simulink model "walkingRobotRL3D"  (R2020b)
settings: Solver=ode23t  StartTime=0.0  StopTime=Tf  RelTol=1e-2  EnableMultiTasking=on
PreLoadFcn:
  | robotParametersRL
undefined symbols (not defined in the file): agent, ankleD_pitch_jointMAX, ankleD_pitch_jointMIN, ankleD_roll_jointMAX, ankleD_roll_jointMIN, ankleI_pitch_jointMAX, ankleI_pitch_jointMIN, ankleI_roll_jointMAX, ankleI_roll_jointMIN, getSampleTime, height_plane, hipD_pitch_jointMAX, hipD_pitch_jointMIN, hipD_roll_jointMAX, hipD_roll_jointMIN, hipI_pitch_jointMAX, hipI_pitch_jointMIN, hipI_roll_jointMAX, hipI_roll_jointMIN, init_angs_L, init_angs_R, init_height, joint_damping, joint_limit_damping, joint_limit_stiffness, joint_stiffness, kneeD_jointMAX, kneeD_jointMIN, kneeI_jointMAX, kneeI_jointMIN, lower_leg_I0, lower_leg_length, lower_leg_mass, lower_leg_x, lower_leg_y, muscle_nominal_length, p10_ankleD_roll, plane_x, plane_y, regulator_type, tau, Tf, torso_height, torso_length, torso_offset_x, torso_offset_z, torso_width, torso_x, torso_y, torso_z, Ts, upper_leg_I0, upper_leg_length, upper_leg_mass, upper_leg_x, upper_leg_y, v10_ankleD_pitch, v10_ankleD_roll, v10_ankleI_pitch, v10_ankleI_roll ... (+41)
libraries: sm_lib x222, simulink x183, nesl_utility x130, walkingRobotUtils x69, rllib x2
(part 21 of 24)

== matlab function walkingRobotRL3D/Walking Robot/DYNAMIC MODEL OF PAM FOR RIGHT LEG/Dynamic Model Antagonisitic PAM2/Proportional Regulator (Muscles 1) ==
  data: V1 input; reg_type input; p1 output
% Author: Eduardo Reyero Ibáñez
% Descrition: In this file it will be implemented the required input for the PAM
function p1  = propReg(V1,reg_type)
%% Proportional pressure regulators VPPM
%Range of Voltage
minVoltage = 0;
maxVoltage = 7.98; % This voltage provide 8 bar of pressure with regulator type 1
p1 = zeros(1,1);
%Select regulartor type
%reg_type = 1; % This will be given by the call of the function
%Limit the voltage
for i=1:length(p1)
if V1(i) >= maxVoltage 
    V1(i) = maxVoltage;
end
end
if reg_type == 1
    f_prop = @(V) 0.99*V+0.1;
    for i=1:length(p1)
    p1(i) = f_prop(V1(i));
    end
elseif reg_type == 2
    f_prop = @(V) 0.594*V+0.06;
    for i=1:length(p1)
    p1(i) = f_prop(V1(i));
    end
else
    f_prop = @(V) 0.198*V+0.02;
    for i=1:length(p1)
    p1(i) = f_prop(V1(i));
    end
end

% figure
% fplot(p1)
% xlim([0 10])
% ylim([0 10])
end

== matlab function walkingRobotRL3D/Walking Robot/DYNAMIC MODEL OF PAM FOR RIGHT LEG/Dynamic Model Antagonisitic PAM2/Proportional Regulator (Muscles 2) ==
  data: V1 input; reg_type input; p1 output
% Author: Eduardo Reyero Ibáñez
% Descrition: In this file it will be implemented the required input for the PAM
function p1  = propReg(V1,reg_type)
%% Proportional pressure regulators VPPM
%Range of Voltage
minVoltage = 0;
maxVoltage = 7.98; % This voltage provide 8 bar of pressure with regulator type 1
p1 = zeros(1,1);
%Select regulartor type
%reg_type = 1; % This will be given by the call of the function
%Limit the voltage
for i=1:length(p1)
if V1(i) >= maxVoltage 
    V1(i) = maxVoltage;
end
end
if reg_type == 1
    f_prop = @(V) 0.99*V+0.1;
    for i=1:length(p1)
    p1(i) = f_prop(V1(i));
    end
elseif reg_type == 2
    f_prop = @(V) 0.594*V+0.06;
    for i=1:length(p1)
    p1(i) = f_prop(V1(i));
    end
else
    f_prop = @(V) 0.198*V+0.02;
    for i=1:length(p1)
    p1(i) = f_prop(V1(i));
    end
end

% figure
% fplot(p1)
% xlim([0 10])
% ylim([0 10])
end

== matlab function walkingRobotRL3D/Walking Robot/DYNAMIC MODEL OF PAM FOR RIGHT LEG/Dynamic Model Antagonisitic PAM2/Spring and damping model/S(P),D(P) ==
  data: P1 input; S1 output; P2 input; D1 output; S2 output; D2 output
function [S1,D1,S2,D2] = getSpringDampingCoeff(P1,P2)
tau = 0.6;
% Spring and damping coeff for muscle 1
if P1>=0 && P1<=1
    S1 = 400;
    D1 = tau*S1;
elseif P1>1 && P1<=2
    S1 = 500;
    D1 = tau*S1;
elseif P1>2 && P1<=3
    S1 = 1100;
    D1 = tau*S1;
elseif P1>3 && P1<=4
    S1 = 1500;
    D1 = tau*S1;
elseif P1>4 && P1<=5
    S1 = 2000;
    D1 = tau*S1;
elseif P1>5 && P1<=6
    S1 = 2900;
    D1 = tau*S1;
elseif P1>6 && P1<=7
    S1 = 3800;
    D1 = tau*S1;
elseif P1>7 && P1<=8.5
    S1 = 5000;
    D1 = tau*S1;
else %Never will enter here
    S1 = 800;
    D1 = tau*S1;  
end

% Spring and damping coeff for muscle 1
if P2>=0 && P2<=1
    S2 = 400;
    D2 = tau*S2;
elseif P2>1 && P2<=2
    S2 = 500;
    D2 = tau*S2;
elseif P2>2 && P2<=3
    S2 = 1100;
    D2 = tau*S2;
elseif P2>3 && P2<=4
    S2 = 1500;
    D2 = tau*S2;
elseif P2>4 && P2<=5
    S2 = 2000;
    D2 = tau*S2;
elseif P2>5 && P2<=6
    S2 = 2900;
    D2 = tau*S2;
elseif P2>6 && P2<=7
    S2 = 3800;
    D2 = tau*S2;
elseif P2>7 && P2<=8.5
    S2 = 5000;
    D2 = tau*S2;
else %Never will enter here
    S2 = 800;
    D2 = tau*S2;  
end

end

== matlab function walkingRobotRL3D/Walking Robot (Angle based)/Dynamic model of antagonistic PAM actuators/F(x,P) mode (Muscles 1) ==
  data: P1 input; F1 output; x_muscle1 input
%Author: Eduardo Reyero Ibáñez
%Note: F(x) curves for different pressures are limited by recommended
%limitation of 20% in contraction percentage for the used PAM actuator
%(L = 260mm D=20mm)
function F1 = FxPmodel(P1,x_muscle1)
%Input: P comming from proporcional controller  is in bar. Its 6x1 vector
% x_muscle (in % contraction)
%Output:F according to P input and and x value of half of the maximun
%permissible stroke
%Importing 2 variable F(x,P) model
curve = @(x,P)  -0.002697-93.8*x+2.917*P+13.05*x^2-0.04264*x*P-0.001793*P^2-0.9395*x^3-0.001597*x^2*P-0.0001142*x*P^2+4.694e-06*P^3+0.03335*x^4+6.106e-06*x^3*P+2.699e-06*x^2*P^2+1.25e-07*x*P^3-5.675e-09*P^4-0.0004611*x^5+9.334e-07*x^4*P-1.221e-08*x^3*P^2-1.463e-09*x^2*P^3-4.929e-11*x*P^4+2.492e-12*P^5;
%Defining F and x vectors for the 6 actuators
F1 = zeros(length(P1),1); %6x1
x1 = zeros(length(P1),1); %6x1
% Transform P from bar to Kpa
P1 = 100*P1;

for i=1:length(P1)
% Obtaining the stroke
x1(i) = x_muscle1(i); 
% Obtaining the applied force
F1(i) = curve(x1(i),P1(i)); 
end
end

== matlab function walkingRobotRL3D/Walking Robot/DYNAMIC MODEL OF PAM FOR RIGHT LEG/Dynamic Model Antagonisitic PAM3/F(x,P) mode (Muscles 1) ==
  data: P1 input; F1 output; x_muscle1 input
%Author: Eduardo Reyero Ibáñez
%Note: F(x) curves for different pressures are limited by recommended
%limitation of 20% in contraction percentage for the used PAM actuator
%(L = 260mm D=20mm)
function F1 = FxPmodel(P1,x_muscle1)
%Input: P comming from proporcional controller  is in bar. Its 6x1 vector
% x_muscle (in % contraction)
%Output:F according to P input and and x value of half of the maximun
%permissible stroke
%Importing 2 variable F(x,P) model
curve = @(x,P)  -0.002697-93.8*x+2.917*P+13.05*x^2-0.04264*x*P-0.001793*P^2-0.9395*x^3-0.001597*x^2*P-0.0001142*x*P^2+4.694e-06*P^3+0.03335*x^4+6.106e-06*x^3*P+2.699e-06*x^2*P^2+1.25e-07*x*P^3-5.675e-09*P^4-0.0004611*x^5+9.334e-07*x^4*P-1.221e-08*x^3*P^2-1.463e-09*x^2*P^3-4.929e-11*x*P^4+2.492e-12*P^5;
%Defining F and x vectors for the 6 actuators
F1 = zeros(length(P1),1); %6x1
x1 = zeros(length(P1),1); %6x1
% Transform P from bar to Kpa
P1 = 100*P1;

for i=1:length(P1)
% Obtaining the stroke
x1(i) = x_muscle1(i); 
% Obtaining the applied force
F1(i) = curve(x1(i),P1(i)); 
if F1(i)<0
    F1(i) = 0;
end
end
end

== matlab function walkingRobotRL3D/Walking Robot/DYNAMIC MODEL OF PAM FOR RIGHT LEG/Dynamic Model Antagonisitic PAM3/F(x,P) mode (Muscles 1)1 ==
  data: P2 input; F2 output; x_muscle2 input
%Author: Eduardo Reyero Ibáñez
%Note: F(x) curves for different pressures are limited by recommended
%limitation of 20% in contraction percentage for the used PAM actuator
%(L = 260mm D=20mm)
function F2 = FxPmodel(P2,x_muscle2)
%Input: P comming from proporcional controller  is in bar. Its 6x1 vector
% x_muscle (in % contraction)
%Output:F according to P input and and x value of half of the maximun
%permissible stroke
%Importing 2 variable F(x,P) model
curve = @(x,P)  -0.002697-93.8*x+2.917*P+13.05*x^2-0.04264*x*P-0.001793*P^2-0.9395*x^3-0.001597*x^2*P-0.0001142*x*P^2+4.694e-06*P^3+0.03335*x^4+6.106e-06*x^3*P+2.699e-06*x^2*P^2+1.25e-07*x*P^3-5.675e-09*P^4-0.0004611*x^5+9.334e-07*x^4*P-1.221e-08*x^3*P^2-1.463e-09*x^2*P^3-4.929e-11*x*P^4+2.492e-12*P^5;
%Defining F and x vectors for the 6 actuators
F2 = zeros(length(P2),1); %6x1
x2 = zeros(length(P2),1); %6x1
% Transform P from bar to Kpa
P2 = 100*P2;

for i=1:length(P2)
% Obtaining the stroke
x2(i) = x_muscle2(i); 
% Obtaining the applied force
F2(i) = curve(x2(i),P2(i));
if F2(i)<0
    F2(i) = 0;
end
end
end

== matlab function walkingRobotRL3D/Walking Robot/DYNAMIC MODEL OF PAM FOR RIGHT LEG/Dynamic Model Antagonisitic PAM3/Proportional Regulator (Muscles 1) ==
  data: V1 input; reg_type input; p1 output
% Author: Eduardo Reyero Ibáñez
% Descrition: In this file it will be implemented the required input for the PAM
function p1  = propReg(V1,reg_type)
%% Proportional pressure regulators VPPM
%Range of Voltage
minVoltage = 0;
maxVoltage = 7.98; % This voltage provide 8 bar of pressure with regulator type 1
p1 = zeros(1,1);
%Select regulartor type
%reg_type = 1; % This will be given by the call of the function
%Limit the voltage
for i=1:length(p1)
if V1(i) >= maxVoltage 
    V1(i) = maxVoltage;
end
end
if reg_type == 1
    f_prop = @(V) 0.99*V+0.1;
    for i=1:length(p1)
    p1(i) = f_prop(V1(i));
    end
elseif reg_type == 2
    f_prop = @(V) 0.594*V+0.06;
    for i=1:length(p1)
    p1(i) = f_prop(V1(i));
    end
else
    f_prop = @(V) 0.198*V+0.02;
    for i=1:length(p1)
    p1(i) = f_prop(V1(i));
    end
end

% figure
% fplot(p1)
% xlim([0 10])
% ylim([0 10])
end

== matlab function walkingRobotRL3D/Walking Robot/DYNAMIC MODEL OF PAM FOR RIGHT LEG/Dynamic Model Antagonisitic PAM3/Proportional Regulator (Muscles 2) ==
  data: V1 input; reg_type input; p1 output
% Author: Eduardo Reyero Ibáñez
% Descrition: In this file it will be implemented the required input for the PAM
function p1  = propReg(V1,reg_type)
%% Proportional pressure regulators VPPM
%Range of Voltage
minVoltage = 0;
maxVoltage = 7.98; % This voltage provide 8 bar of pressure with regulator type 1
p1 = zeros(1,1);
%Select regulartor type
%reg_type = 1; % This will be given by the call of the function
%Limit the voltage
for i=1:length(p1)
if V1(i) >= maxVoltage 
    V1(i) = maxVoltage;
end
end
if reg_type == 1
    f_prop = @(V) 0.99*V+0.1;
    for i=1:length(p1)
    p1(i) = f_prop(V1(i));
    end
elseif reg_type == 2
    f_prop = @(V) 0.594*V+0.06;
    for i=1:length(p1)
    p1(i) = f_prop(V1(i));
    end
else
    f_prop = @(V) 0.198*V+0.02;
    for i=1:length(p1)
    p1(i) = f_prop(V1(i));
    end
end

% figure
% fplot(p1)
% xlim([0 10])
% ylim([0 10])
end

== matlab function walkingRobotRL3D/Walking Robot/DYNAMIC MODEL OF PAM FOR RIGHT LEG/Dynamic Model Antagonisitic PAM3/Spring and damping model/S(P),D(P) ==
  data: P1 input; S1 output; P2 input; D1 output; S2 output; D2 output
function [S1,D1,S2,D2] = getSpringDampingCoeff(P1,P2)
tau = 0.6;
% Spring and damping coeff for muscle 1
if P1>=0 && P1<=1
    S1 = 400;
    D1 = tau*S1;
elseif P1>1 && P1<=2
    S1 = 500;
    D1 = tau*S1;
elseif P1>2 && P1<=3
    S1 = 1100;
    D1 = tau*S1;
elseif P1>3 && P1<=4
    S1 = 1500;
    D1 = tau*S1;
elseif P1>4 && P1<=5
    S1 = 2000;
    D1 = tau*S1;
elseif P1>5 && P1<=6
    S1 = 2900;
    D1 = tau*S1;
elseif P1>6 && P1<=7
    S1 = 3800;
    D1 = tau*S1;
elseif P1>7 && P1<=8.5
    S1 = 5000;
    D1 = tau*S1;
else %Never will enter here
    S1 = 800;
    D1 = tau*S1;  
end

% Spring and damping coeff for muscle 1
if P2>=0 && P2<=1
    S2 = 400;
    D2 = tau*S2;
elseif P2>1 && P2<=2
    S2 = 500;
    D2 = tau*S2;
elseif P2>2 && P2<=3
    S2 = 1100;
    D2 = tau*S2;
elseif P2>3 && P2<=4
    S2 = 1500;
    D2 = tau*S2;
elseif P2>4 && P2<=5
    S2 = 2000;
    D2 = tau*S2;
elseif P2>5 && P2<=6
    S2 = 2900;
    D2 = tau*S2;
elseif P2>6 && P2<=7
    S2 = 3800;
    D2 = tau*S2;
elseif P2>7 && P2<=8.5
    S2 = 5000;
    D2 = tau*S2;
else %Never will enter here
    S2 = 800;
    D2 = tau*S2;  
end

end

== matlab function walkingRobotRL3D/Walking Robot/DYNAMIC MODEL OF PAM FOR RIGHT LEG/Dynamic Model Antagonisitic PAM4/F(x,P) mode (Muscles 1) ==
  data: P1 input; F1 output; x_muscle1 input
%Author: Eduardo Reyero Ibáñez
%Note: F(x) curves for different pressures are limited by recommended
%limitation of 20% in contraction percentage for the used PAM actuator
%(L = 260mm D=20mm)
function F1 = FxPmodel(P1,x_muscle1)
%Input: P comming from proporcional controller  is in bar. Its 6x1 vector
% x_muscle (in % contraction)
%Output:F according to P input and and x value of half of the maximun
%permissible stroke
%Importing 2 variable F(x,P) model
curve = @(x,P)  -0.002697-93.8*x+2.917*P+13.05*x^2-0.04264*x*P-0.001793*P^2-0.9395*x^3-0.001597*x^2*P-0.0001142*x*P^2+4.694e-06*P^3+0.03335*x^4+6.106e-06*x^3*P+2.699e-06*x^2*P^2+1.25e-07*x*P^3-5.675e-09*P^4-0.0004611*x^5+9.334e-07*x^4*P-1.221e-08*x^3*P^2-1.463e-09*x^2*P^3-4.929e-11*x*P^4+2.492e-12*P^5;
%Defining F and x vectors for the 6 actuators
F1 = zeros(length(P1),1); %6x1
x1 = zeros(length(P1),1); %6x1
% Transform P from bar to Kpa
P1 = 100*P1;

for i=1:length(P1)
% Obtaining the stroke
x1(i) = x_muscle1(i); 
% Obtaining the applied force
F1(i) = curve(x1(i),P1(i)); 
if F1(i)<0
    F1(i) = 0;
end
end
end

== matlab function walkingRobotRL3D/Walking Robot/DYNAMIC MODEL OF PAM FOR RIGHT LEG/Dynamic Model Antagonisitic PAM4/F(x,P) mode (Muscles 1)1 ==
  data: P2 input; F2 output; x_muscle2 input
%Author: Eduardo Reyero Ibáñez
%Note: F(x) curves for different pressures are limited by recommended
%limitation of 20% in contraction percentage for the used PAM actuator
%(L = 260mm D=20mm)
function F2 = FxPmodel(P2,x_muscle2)
%Input: P comming from proporcional controller  is in bar. Its 6x1 vector
% x_muscle (in % contraction)
%Output:F according to P input and and x value of half of the maximun
%permissible stroke
%Importing 2 variable F(x,P) model
curve = @(x,P)  -0.002697-93.8*x+2.917*P+13.05*x^2-0.04264*x*P-0.001793*P^2-0.9395*x^3-0.001597*x^2*P-0.0001142*x*P^2+4.694e-06*P^3+0.03335*x^4+6.106e-06*x^3*P+2.699e-06*x^2*P^2+1.25e-07*x*P^3-5.675e-09*P^4-0.0004611*x^5+9.334e-07*x^4*P-1.221e-08*x^3*P^2-1.463e-09*x^2*P^3-4.929e-11*x*P^4+2.492e-12*P^5;
%Defining F and x vectors for the 6 actuators
F2 = zeros(length(P2),1); %6x1
x2 = zeros(length(P2),1); %6x1
% Transform P from bar to Kpa
P2 = 100*P2;

for i=1:length(P2)
% Obtaining the stroke
x2(i) = x_muscle2(i); 
% Obtaining the applied force
F2(i) = curve(x2(i),P2(i));
if F2(i)<0
    F2(i) = 0;
end
end
end

== matlab function walkingRobotRL3D/Walking Robot/DYNAMIC MODEL OF PAM FOR RIGHT LEG/Dynamic Model Antagonisitic PAM4/Proportional Regulator (Muscles 1) ==
  data: V1 input; reg_type input; p1 output
% Author: Eduardo Reyero Ibáñez
% Descrition: In this file it will be implemented the required input for the PAM
function p1  = propReg(V1,reg_type)
%% Proportional pressure regulators VPPM
%Range of Voltage
minVoltage = 0;
maxVoltage = 7.98; % This voltage provide 8 bar of pressure with regulator type 1
p1 = zeros(1,1);
%Select regulartor type
%reg_type = 1; % This will be given by the call of the function
%Limit the voltage
for i=1:length(p1)
if V1(i) >= maxVoltage 
    V1(i) = maxVoltage;
end
end
if reg_type == 1
    f_prop = @(V) 0.99*V+0.1;
    for i=1:length(p1)
    p1(i) = f_prop(V1(i));
    end
elseif reg_type == 2
    f_prop = @(V) 0.594*V+0.06;
    for i=1:length(p1)
    p1(i) = f_prop(V1(i));
    end
else
    f_prop = @(V) 0.198*V+0.02;
    for i=1:length(p1)
    p1(i) = f_prop(V1(i));
    end
end

% figure
% fplot(p1)
% xlim([0 10])
% ylim([0 10])
end

== matlab function walkingRobotRL3D/Walking Robot/DYNAMIC MODEL OF PAM FOR RIGHT LEG/Dynamic Model Antagonisitic PAM4/Proportional Regulator (Muscles 2) ==
  data: V1 input; reg_type input; p1 output
% Author: Eduardo Reyero Ibáñez
% Descrition: In this file it will be implemented the required input for the PAM
function p1  = propReg(V1,reg_type)
%% Proportional pressure regulators VPPM
%Range of Voltage
minVoltage = 0;
maxVoltage = 7.98; % This voltage provide 8 bar of pressure with regulator type 1
p1 = zeros(1,1);
%Select regulartor type
%reg_type = 1; % This will be given by the call of the function
%Limit the voltage
for i=1:length(p1)
if V1(i) >= maxVoltage 
    V1(i) = maxVoltage;
end
end
if reg_type == 1
    f_prop = @(V) 0.99*V+0.1;
    for i=1:length(p1)
    p1(i) = f_prop(V1(i));
    end
elseif reg_type == 2
    f_prop = @(V) 0.594*V+0.06;
    for i=1:length(p1)
    p1(i) = f_prop(V1(i));
    end
else
    f_prop = @(V) 0.198*V+0.02;
    for i=1:length(p1)
    p1(i) = f_prop(V1(i));
    end
end

% figure
% fplot(p1)
% xlim([0 10])
% ylim([0 10])
end

== matlab function walkingRobotRL3D/Walking Robot (Angle based)/Dynamic model of antagonistic PAM actuators/F(x,P) model1 (Muscles 2) ==
  data: P2 input; F2 output; x_muscle2 input
%Author: Eduardo Reyero Ibáñez
%Note: F(x) curves for different pressures are limited by recommended
%limitation of 20% in contraction percentage for the used PAM actuator
%(L = 260mm D=20mm)
function F2 = FxPmodel(P2,x_muscle2)
%Input: P comming from proporcional controller  is in bar. Its 6x1 vector
% x_muscle2 in (% contraction)
%Output:F according to P input and and x value of half of the maximun
%permissible stroke
%Importing 2 variable F(x,P) model
curve = @(x,P)  -0.002697-93.8*x+2.917*P+13.05*x^2-0.04264*x*P-0.001793*P^2-0.9395*x^3-0.001597*x^2*P-0.0001142*x*P^2+4.694e-06*P^3+0.03335*x^4+6.106e-06*x^3*P+2.699e-06*x^2*P^2+1.25e-07*x*P^3-5.675e-09*P^4-0.0004611*x^5+9.334e-07*x^4*P-1.221e-08*x^3*P^2-1.463e-09*x^2*P^3-4.929e-11*x*P^4+2.492e-12*P^5;

%Defining F and x vectors for the 6 actuators
F2 = zeros(length(P2),1); %6x1
x2 = zeros(length(P2),1); %6x1
%x2 = [14.06 28.12 14.06 14.06 28.12 14.06]';
% Transform P from bar to Kpa
P2 = 100*P2;

for i=1:length(P2)
% Obtaining the stroke max/2
x2(i) = x_muscle2(i); 
% Obtaining the applied force
F2(i) = curve(x2(i),P2(i)); 
end
end

== matlab function walkingRobotRL3D/Walking Robot/DYNAMIC MODEL OF PAM FOR RIGHT LEG/Dynamic Model Antagonisitic PAM4/Spring and damping model/S(P),D(P) ==
  data: P1 input; S1 output; P2 input; D1 output; S2 output; D2 output
function [S1,D1,S2,D2] = getSpringDampingCoeff(P1,P2)
tau = 0.6;
% Spring and damping coeff for muscle 1
if P1>=0 && P1<=1
    S1 = 400;
    D1 = tau*S1;
elseif P1>1 && P1<=2
    S1 = 500;
    D1 = tau*S1;
elseif P1>2 && P1<=3
    S1 = 1100;
    D1 = tau*S1;
elseif P1>3 && P1<=4
    S1 = 1500;
    D1 = tau*S1;
elseif P1>4 && P1<=5
    S1 = 2000;
    D1 = tau*S1;
elseif P1>5 && P1<=6
    S1 = 2900;
    D1 = tau*S1;
elseif P1>6 && P1<=7
    S1 = 3800;
    D1 = tau*S1;
elseif P1>7 && P1<=8.5
    S1 = 5000;
    D1 = tau*S1;
else %Never will enter here
    S1 = 800;
    D1 = tau*S1;  
end

% Spring and damping coeff for muscle 1
if P2>=0 && P2<=1
    S2 = 400;
    D2 = tau*S2;
elseif P2>1 && P2<=2
    S2 = 500;
    D2 = tau*S2;
elseif P2>2 && P2<=3
    S2 = 1100;
    D2 = tau*S2;
elseif P2>3 && P2<=4
    S2 = 1500;
    D2 = tau*S2;
elseif P2>4 && P2<=5
    S2 = 2000;
    D2 = tau*S2;
elseif P2>5 && P2<=6
    S2 = 2900;
    D2 = tau*S2;
elseif P2>6 && P2<=7
    S2 = 3800;
    D2 = tau*S2;
elseif P2>7 && P2<=8.5
    S2 = 5000;
    D2 = tau*S2;
else %Never will enter here
    S2 = 800;
    D2 = tau*S2;  
end

end

== matlab function walkingRobotRL3D/Walking Robot/DYNAMIC MODEL OF PAM FOR RIGHT LEG/Dynamic Model Antagonisitic PAM5/F(x,P) mode (Muscles 1) ==
  data: P1 input; F1 output; x_muscle1 input
%Author: Eduardo Reyero Ibáñez
%Note: F(x) curves for different pressures are limited by recommended
%limitation of 20% in contraction percentage for the used PAM actuator
%(L = 260mm D=20mm)
function F1 = FxPmodel(P1,x_muscle1)
%Input: P comming from proporcional controller  is in bar. Its 6x1 vector
% x_muscle (in % contraction)
%Output:F according to P input and and x value of half of the maximun
%permissible stroke
%Importing 2 variable F(x,P) model
curve = @(x,P)  -0.002697-93.8*x+2.917*P+13.05*x^2-0.04264*x*P-0.001793*P^2-0.9395*x^3-0.001597*x^2*P-0.0001142*x*P^2+4.694e-06*P^3+0.03335*x^4+6.106e-06*x^3*P+2.699e-06*x^2*P^2+1.25e-07*x*P^3-5.675e-09*P^4-0.0004611*x^5+9.334e-07*x^4*P-1.221e-08*x^3*P^2-1.463e-09*x^2*P^3-4.929e-11*x*P^4+2.492e-12*P^5;
%Defining F and x vectors for the 6 actuators
F1 = zeros(length(P1),1); %6x1
x1 = zeros(length(P1),1); %6x1
% Transform P from bar to Kpa
P1 = 100*P1;

for i=1:length(P1)
% Obtaining the stroke
x1(i) = x_muscle1(i); 
% Obtaining the applied force
F1(i) = curve(x1(i),P1(i)); 
if F1(i)<0
    F1(i) = 0;
end
end
end

== matlab function walkingRobotRL3D/Walking Robot/DYNAMIC MODEL OF PAM FOR RIGHT LEG/Dynamic Model Antagonisitic PAM5/F(x,P) mode (Muscles 1)1 ==
  data: P2 input; F2 output; x_muscle2 input
%Author: Eduardo Reyero Ibáñez
%Note: F(x) curves for different pressures are limited by recommended
%limitation of 20% in contraction percentage for the used PAM actuator
%(L = 260mm D=20mm)
function F2 = FxPmodel(P2,x_muscle2)
%Input: P comming from proporcional controller  is in bar. Its 6x1 vector
% x_muscle (in % contraction)
%Output:F according to P input and and x value of half of the maximun
%permissible stroke
%Importing 2 variable F(x,P) model
curve = @(x,P)  -0.002697-93.8*x+2.917*P+13.05*x^2-0.04264*x*P-0.001793*P^2-0.9395*x^3-0.001597*x^2*P-0.0001142*x*P^2+4.694e-06*P^3+0.03335*x^4+6.106e-06*x^3*P+2.699e-06*x^2*P^2+1.25e-07*x*P^3-5.675e-09*P^4-0.0004611*x^5+9.334e-07*x^4*P-1.221e-08*x^3*P^2-1.463e-09*x^2*P^3-4.929e-11*x*P^4+2.492e-12*P^5;
%Defining F and x vectors for the 6 actuators
F2 = zeros(length(P2),1); %6x1
x2 = zeros(length(P2),1); %6x1
% Transform P from bar to Kpa
P2 = 100*P2;

for i=1:length(P2)
% Obtaining the stroke
x2(i) = x_muscle2(i); 
% Obtaining the applied force
F2(i) = curve(x2(i),P2(i));
if F2(i)<0
    F2(i) = 0;
end
end
end

== matlab function walkingRobotRL3D/Walking Robot/DYNAMIC MODEL OF PAM FOR RIGHT LEG/Dynamic Model Antagonisitic PAM5/Proportional Regulator (Muscles 1) ==
  data: V1 input; reg_type input; p1 output
% Author: Eduardo Reyero Ibáñez
% Descrition: In this file it will be implemented the required input for the PAM
function p1  = propReg(V1,reg_type)
%% Proportional pressure regulators VPPM
%Range of Voltage
minVoltage = 0;
maxVoltage = 7.98; % This voltage provide 8 bar of pressure with regulator type 1
p1 = zeros(1,1);
%Select regulartor type
%reg_type = 1; % This will be given by the call of the function
%Limit the voltage
for i=1:length(p1)
if V1(i) >= maxVoltage 
    V1(i) = maxVoltage;
end
end
if reg_type == 1
    f_prop = @(V) 0.99*V+0.1;
    for i=1:length(p1)
    p1(i) = f_prop(V1(i));
    end
elseif reg_type == 2
    f_prop = @(V) 0.594*V+0.06;
    for i=1:length(p1)
    p1(i) = f_prop(V1(i));
    end
else
    f_prop = @(V) 0.198*V+0.02;
    for i=1:length(p1)
    p1(i) = f_prop(V1(i));
    end
end

% figure
% fplot(p1)
% xlim([0 10])
% ylim([0 10])
end

== matlab function walkingRobotRL3D/Walking Robot/DYNAMIC MODEL OF PAM FOR RIGHT LEG/Dynamic Model Antagonisitic PAM5/Proportional Regulator (Muscles 2) ==
  data: V1 input; reg_type input; p1 output
% Author: Eduardo Reyero Ibáñez
% Descrition: In this file it will be implemented the required input for the PAM
function p1  = propReg(V1,reg_type)
%% Proportional pressure regulators VPPM
%Range of Voltage
minVoltage = 0;
maxVoltage = 7.98; % This voltage provide 8 bar of pressure with regulator type 1
p1 = zeros(1,1);
%Select regulartor type
%reg_type = 1; % This will be given by the call of the function
%Limit the voltage
for i=1:length(p1)
if V1(i) >= maxVoltage 
    V1(i) = maxVoltage;
end
end
if reg_type == 1
    f_prop = @(V) 0.99*V+0.1;
    for i=1:length(p1)
    p1(i) = f_prop(V1(i));
    end
elseif reg_type == 2
    f_prop = @(V) 0.594*V+0.06;
    for i=1:length(p1)
    p1(i) = f_prop(V1(i));
    end
else
    f_prop = @(V) 0.198*V+0.02;
    for i=1:length(p1)
    p1(i) = f_prop(V1(i));
    end
end

% figure
% fplot(p1)
% xlim([0 10])
% ylim([0 10])
end

== matlab function walkingRobotRL3D/Walking Robot/DYNAMIC MODEL OF PAM FOR RIGHT LEG/Dynamic Model Antagonisitic PAM5/Spring and damping model/S(P),D(P) ==
  data: P1 input; S1 output; P2 input; D1 output; S2 output; D2 output
function [S1,D1,S2,D2] = getSpringDampingCoeff(P1,P2)
tau = 0.6;
% Spring and damping coeff for muscle 1
if P1>=0 && P1<=1
    S1 = 400;
    D1 = tau*S1;
elseif P1>1 && P1<=2
    S1 = 500;
    D1 = tau*S1;
elseif P1>2 && P1<=3
    S1 = 1100;
    D1 = tau*S1;
elseif P1>3 && P1<=4
    S1 = 1500;
    D1 = tau*S1;
elseif P1>4 && P1<=5
    S1 = 2000;
    D1 = tau*S1;
elseif P1>5 && P1<=6
    S1 = 2900;
    D1 = tau*S1;
elseif P1>6 && P1<=7
    S1 = 3800;
    D1 = tau*S1;
elseif P1>7 && P1<=8.5
    S1 = 5000;
    D1 = tau*S1;
else %Never will enter here
    S1 = 800;
    D1 = tau*S1;  
end

% Spring and damping coeff for muscle 1
if P2>=0 && P2<=1
    S2 = 400;
    D2 = tau*S2;
elseif P2>1 && P2<=2
    S2 = 500;
    D2 = tau*S2;
elseif P2>2 && P2<=3
    S2 = 1100;
    D2 = tau*S2;
elseif P2>3 && P2<=4
    S2 = 1500;
    D2 = tau*S2;
elseif P2>4 && P2<=5
    S2 = 2000;
    D2 = tau*S2;
elseif P2>5 && P2<=6
    S2 = 2900;
    D2 = tau*S2;
elseif P2>6 && P2<=7
    S2 = 3800;
    D2 = tau*S2;
elseif P2>7 && P2<=8.5
    S2 = 5000;
    D2 = tau*S2;
else %Never will enter here
    S2 = 800;
    D2 = tau*S2;  
end

end

== matlab function walkingRobotRL3D/Walking Robot/DYNAMIC MODEL OF PAM FOR RIGHT LEG/F-->Torque1 ==
  data: R1 input; torque output; R2 input
%Author: Eduardo Reyero
%Description: This file provides the Torque to apply to each joint of the
%robot based on the F(x) model input
function torque = getTorque(R1,R2)
%Define function
torque = zeros(length(R1),1);
%Defining radius of the pulleys (m) (define values when know them)
pulley_radius = 0.03; %(m) 
torque(1) = (R1(1)-R2(1))*pulley_radius;
%Torque is calcultad as T = (F1-F2)*r
% Para los del tobillo seria algo como F1(x1-x10) - F2(x2-x20)
end

== matlab function walkingRobotRL3D/Walking Robot/DYNAMIC MODEL OF PAM FOR RIGHT LEG/F-->Torque2 ==
  data: R1 input; torque output; R2 input
%Author: Eduardo Reyero
%Description: This file provides the Torque to apply to each joint of the
%robot based on the F(x) model input
function torque = getTorque(R1,R2)
%Define function
torque = zeros(length(R1),1);
%Defining radius of the pulleys (m) (define values when know them)
pulley_radius = 0.05; %(m) 
torque(1) = (R1(1)-R2(1))*pulley_radius;
%Torque is calcultad as T = (F1-F2)*r
% Para los del tobillo seria algo como F1(x1-x10) - F2(x2-x20)
end

== matlab function walkingRobotRL3D/Walking Robot/DYNAMIC MODEL OF PAM FOR RIGHT LEG/F-->Torque3 ==
  data: R1 input; torque output; R2 input
%Author: Eduardo Reyero
%Description: This file provides the Torque to apply to each joint of the
%robot based on the F(x) model input
function torque = getTorque(R1,R2)
%Define function
torque = zeros(length(R1),1);
%Defining radius of the pulleys (m) (define values when know them)
pulley_radius = 0.03; %(m) 
torque(1) = (R1(1)-R2(1))*pulley_radius;
%Torque is calcultad as T = (F1-F2)*r
% Para los del tobillo seria algo como F1(x1-x10) - F2(x2-x20)
end

== matlab function walkingRobotRL3D/Walking Robot/DYNAMIC MODEL OF PAM FOR RIGHT LEG/F-->Torque4 ==
  data: R1 input; torque output; R2 input
%Author: Eduardo Reyero
%Description: This file provides the Torque to apply to each joint of the
%robot based on the F(x) model input
function torque = getTorque(R1,R2)
%Define function
torque = zeros(length(R1),1);
%Defining radius of the pulleys (m) (define values when know them)
pulley_radius = 0.05; %(m) 
torque(1) = (R1(1)-R2(1))*pulley_radius;
%Torque is calcultad as T = (F1-F2)*r
% Para los del tobillo seria algo como F1(x1-x10) - F2(x2-x20)
end

== matlab function walkingRobotRL3D/Walking Robot (Angle based)/Dynamic model of antagonistic PAM actuators/F-->Torque ==
  data: F1 input; torque output; F2 input
%Author: Eduardo Reyero
%Description: This file provides the Torque to apply to each joint of the
%robot based on the F(x) model input
%Input: Two 10x1 matrix of Forces. First matrix has the F1 forces which
%apply one of the two muscles on each joint. F2 has the forces that applied
%the second muscle on each joint
%Output: 10x1 torque vector(one component for each joint)
function torque = getTorque(F1,F2)
%Define function
torque = zeros(length(F1),1);
%Defining radius of the pulleys (m) (define values when know them)
r_ankle_roll = 0.03;% NOTE: THE ANKLE DOES NOT HAVE THIS MECHANISM.. THINK VARIANT
r_knee = 0.05;
r_hip_roll = 0.05;
r_ankle_pitch = 0.03; % NOTE: THE ANKLE DOES NOT HAVE THIS MECHANISM.. THINK VARIANT
r_hip_pitch = 0.05;

%Torque is calcultad as T = (F1-F2)*r
%Ankle torque
%Roll joint D
torque(1) = (F1(1)-F2(1))*r_ankle_roll;
%Pitch joint D
torque(2) = (F1(2)-F2(2))*r_ankle_pitch;
%Roll joint I  
torque(6) = (F1(6)-F2(6))*r_ankle_roll;
%Pitch joint I  
torque(7) = (F1(7)-F2(7))*r_ankle_pitch;

%Knee torque
%D (Right)
torque(3) = (F1(3)-F2(3))*r_knee;
%I (Left)
torque(8) = (F1(8)-F2(8))*r_knee;
% Hip torque
%Roll joint D
torque(4) = (F1(4)-F2(4))*r_hip_roll;
%Roll joint I
torque(9) = (F1(9)-F2(9))*r_hip_roll;
%Pitch joint D
torque(5) = (F1(5)-F2(5))*r_hip_pitch;
%Pitch joint I
torque(10) = (F1(10)-F2(10))*r_hip_pitch;
end

== matlab function walkingRobotRL3D/Walking Robot/DYNAMIC MODEL OF PAM FOR RIGHT LEG/F-->Torque5 ==
  data: R1 input; torque output; R2 input
%Author: Eduardo Reyero
%Description: This file provides the Torque to apply to each joint of the
%robot based on the F(x) model input
function torque = getTorque(R1,R2)
%Define function
torque = zeros(length(R1),1);
%Defining radius of the pulleys (m) (define values when know them)
pulley_radius = 0.05; %(m) 
torque(1) = (R1(1)-R2(1))*pulley_radius;
%Torque is calcultad as T = (F1-F2)*r
% Para los del tobillo seria algo como F1(x1-x10) - F2(x2-x20)
end

== matlab function walkingRobotRL3D/voltage_to_muscles ==
  data: actions input; mapped_actions output
function mapped_actions = voltage_to_muscles(actions)
%narginchk(20,20)
%nargoutchk(0,20)
% Maps actions from [-1,1] that comes from RL agent to [-0.8,0.8] for the
% muscles
fromLow = -1;
fromHigh= 1;
toLow= -0.8;
toHigh= 0.8;
mapped_actions = (actions - fromLow) .* (toHigh - toLow) ./ (fromHigh - fromLow) + toLow;
end

== matlab function walkingRobotRL3D/Walking Robot1/Dynamic model of antagonistic PAM actuators/Proportional Regulator (Muscles 1) ==
  data: V1 input; reg_type input; p1 output
% Author: Eduardo Reyero Ibáñez
% Descrition: In this file it will be implemented the required input for the PAM
function p1  = propReg(V1,reg_type)
%% Proportional pressure regulators VPPM
%Range of Voltage
minVoltage = 0;
maxVoltage = 7.98; % This voltage provide 8 bar of pressure with regulator type 1
p1 = zeros(10,1);
%Initial pressure for muscles
%p1 = [1.764 0 1.764 1.764 0 1.764]';

%Select regulartor type
%reg_type = 1; % This will be given by the call of the function
%Limit the voltage
for i=1:length(p1)
if V1(i) >= maxVoltage 
    V1(i) = maxVoltage;
end
end
if reg_type == 1
    f_prop = @(V) 0.99*V+0.1;
    for i=1:length(p1)
    p1(i) = f_prop(V1(i));
    end
elseif reg_type == 2
    f_prop = @(V) 0.594*V+0.06;
    for i=1:length(p1)
    p1(i) = f_prop(V1(i));
    end
else
    f_prop = @(V) 0.198*V+0.02;
    for i=1:length(p1)
    p1(i) = f_prop(V1(i));
    end
end

% figure
% fplot(p1)
% xlim([0 10])
% ylim([0 10])
end

== matlab function walkingRobotRL3D/Walking Robot33/DYNAMIC MODEL OF PAM FOR RIGHT LEG/Dynamic Model Antagonisitic PAM1/F(x,P) mode (Muscles 1) ==
  data: P1 input; F1 output; x_muscle1 input
%Author: Eduardo Reyero Ibáñez
%Note: F(x) curves for different pressures are limited by recommended
%limitation of 20% in contraction percentage for the used PAM actuator
%(L = 260mm D=20mm)
function F1 = FxPmodel(P1,x_muscle1)
%Input: P comming from proporcional controller  is in bar. Its 6x1 vector
% x_muscle (in % contraction)
%Output:F according to P input and and x value of half of the maximun
%permissible stroke
%Importing 2 variable F(x,P) model
curve = @(x,P)  -0.002697-93.8*x+2.917*P+13.05*x^2-0.04264*x*P-0.001793*P^2-0.9395*x^3-0.001597*x^2*P-0.0001142*x*P^2+4.694e-06*P^3+0.03335*x^4+6.106e-06*x^3*P+2.699e-06*x^2*P^2+1.25e-07*x*P^3-5.675e-09*P^4-0.0004611*x^5+9.334e-07*x^4*P-1.221e-08*x^3*P^2-1.463e-09*x^2*P^3-4.929e-11*x*P^4+2.492e-12*P^5;
%Defining F and x vectors for the 6 actuators
F1 = zeros(length(P1),1); %6x1
x1 = zeros(length(P1),1); %6x1
% Transform P from bar to Kpa
P1 = 100*P1;

for i=1:length(P1)
% Obtaining the stroke
x1(i) = x_muscle1(i); 
% Obtaining the applied force
F1(i) = curve(x1(i),P1(i)); 
if F1(i)<0
    F1(i) = 0;
end
end
end

== matlab function walkingRobotRL3D/Walking Robot33/DYNAMIC MODEL OF PAM FOR RIGHT LEG/Dynamic Model Antagonisitic PAM1/F(x,P) mode (Muscles 1)1 ==
  data: P2 input; F2 output; x_muscle2 input
%Author: Eduardo Reyero Ibáñez
%Note: F(x) curves for different pressures are limited by recommended
%limitation of 20% in contraction percentage for the used PAM actuator
%(L = 260mm D=20mm)
function F2 = FxPmodel(P2,x_muscle2)
%Input: P comming from proporcional controller  is in bar. Its 6x1 vector
% x_muscle (in % contraction)
%Output:F according to P input and and x value of half of the maximun
%permissible stroke
%Importing 2 variable F(x,P) model
curve = @(x,P)  -0.002697-93.8*x+2.917*P+13.05*x^2-0.04264*x*P-0.001793*P^2-0.9395*x^3-0.001597*x^2*P-0.0001142*x*P^2+4.694e-06*P^3+0.03335*x^4+6.106e-06*x^3*P+2.699e-06*x^2*P^2+1.25e-07*x*P^3-5.675e-09*P^4-0.0004611*x^5+9.334e-07*x^4*P-1.221e-08*x^3*P^2-1.463e-09*x^2*P^3-4.929e-11*x*P^4+2.492e-12*P^5;
%Defining F and x vectors for the 6 actuators
F2 = zeros(length(P2),1); %6x1
x2 = zeros(length(P2),1); %6x1
% Transform P from bar to Kpa
P2 = 100*P2;

for i=1:length(P2)
% Obtaining the stroke
x2(i) = x_muscle2(i); 
% Obtaining the applied force
F2(i) = curve(x2(i),P2(i));
if F2(i)<0
    F2(i) = 0;
end
end
end

== matlab function walkingRobotRL3D/Walking Robot33/DYNAMIC MODEL OF PAM FOR RIGHT LEG/Dynamic Model Antagonisitic PAM1/Proportional Regulator (Muscles 1) ==
  data: V1 input; reg_type input; p1 output
% Author: Eduardo Reyero Ibáñez
% Descrition: In this file it will be implemented the required input for the PAM
function p1  = propReg(V1,reg_type)
%% Proportional pressure regulators VPPM
%Range of Voltage
minVoltage = 0;
maxVoltage = 7.98; % This voltage provide 8 bar of pressure with regulator type 1
p1 = zeros(1,1);
%Select regulartor type
%reg_type = 1; % This will be given by the call of the function
%Limit the voltage
for i=1:length(p1)
if V1(i) >= maxVoltage 
    V1(i) = maxVoltage;
end
end
if reg_type == 1
    f_prop = @(V) 0.99*V+0.1;
    for i=1:length(p1)
    p1(i) = f_prop(V1(i));
    end
elseif reg_type == 2
    f_prop = @(V) 0.594*V+0.06;
    for i=1:length(p1)
    p1(i) = f_prop(V1(i));
    end
else
    f_prop = @(V) 0.198*V+0.02;
    for i=1:length(p1)
    p1(i) = f_prop(V1(i));
    end
end

% figure
% fplot(p1)
% xlim([0 10])
% ylim([0 10])
end

== matlab function walkingRobotRL3D/Walking Robot33/DYNAMIC MODEL OF PAM FOR RIGHT LEG/Dynamic Model Antagonisitic PAM1/Proportional Regulator (Muscles 2) ==
  data: V1 input; reg_type input; p1 output
% Author: Eduardo Reyero Ibáñez
% Descrition: In this file it will be implemented the required input for the PAM
function p1  = propReg(V1,reg_type)
%% Proportional pressure regulators VPPM
%Range of Voltage
minVoltage = 0;
maxVoltage = 7.98; % This voltage provide 8 bar of pressure with regulator type 1
p1 = zeros(1,1);
%Select regulartor type
%reg_type = 1; % This will be given by the call of the function
%Limit the voltage
for i=1:length(p1)
if V1(i) >= maxVoltage 
    V1(i) = maxVoltage;
end
end
if reg_type == 1
    f_prop = @(V) 0.99*V+0.1;
    for i=1:length(p1)
    p1(i) = f_prop(V1(i));
    end
elseif reg_type == 2
    f_prop = @(V) 0.594*V+0.06;
    for i=1:length(p1)
    p1(i) = f_prop(V1(i));
    end
else
    f_prop = @(V) 0.198*V+0.02;
    for i=1:length(p1)
    p1(i) = f_prop(V1(i));
    end
end

% figure
% fplot(p1)
% xlim([0 10])
% ylim([0 10])
end

== matlab function walkingRobotRL3D/Walking Robot33/DYNAMIC MODEL OF PAM FOR RIGHT LEG/Dynamic Model Antagonisitic PAM1/Spring and damping model/S(P),D(P) ==
  data: P1 input; S1 output; P2 input; D1 output; S2 output; D2 output
function [S1,D1,S2,D2] = getSpringDampingCoeff(P1,P2)
tau = 0.6;
% Spring and damping coeff for muscle 1
if P1>=0 && P1<=1
    S1 = 400;
    D1 = tau*S1;
elseif P1>1 && P1<=2
    S1 = 500;
    D1 = tau*S1;
elseif P1>2 && P1<=3
    S1 = 1100;
    D1 = tau*S1;
elseif P1>3 && P1<=4
    S1 = 1500;
    D1 = tau*S1;
elseif P1>4 && P1<=5
    S1 = 2000;
    D1 = tau*S1;
elseif P1>5 && P1<=6
    S1 = 2900;
    D1 = tau*S1;
elseif P1>6 && P1<=7
    S1 = 3800;
    D1 = tau*S1;
elseif P1>7 && P1<=8.5
    S1 = 5000;
    D1 = tau*S1;
else %Never will enter here
    S1 = 800;
    D1 = tau*S1;  
end

% Spring and damping coeff for muscle 1
if P2>=0 && P2<=1
    S2 = 400;
    D2 = tau*S2;
elseif P2>1 && P2<=2
    S2 = 500;
    D2 = tau*S2;
elseif P2>2 && P2<=3
    S2 = 1100;
    D2 = tau*S2;
elseif P2>3 && P2<=4
    S2 = 1500;
    D2 = tau*S2;
elseif P2>4 && P2<=5
    S2 = 2000;
    D2 = tau*S2;
elseif P2>5 && P2<=6
    S2 = 2900;
    D2 = tau*S2;
elseif P2>6 && P2<=7
    S2 = 3800;
    D2 = tau*S2;
elseif P2>7 && P2<=8.5
    S2 = 5000;
    D2 = tau*S2;
else %Never will enter here
    S2 = 800;
    D2 = tau*S2;  
end

end

== matlab function walkingRobotRL3D/Walking Robot33/DYNAMIC MODEL OF PAM FOR RIGHT LEG/Dynamic Model Antagonisitic PAM2/F(x,P) mode (Muscles 1) ==
  data: P1 input; F1 output; x_muscle1 input
%Author: Eduardo Reyero Ibáñez
%Note: F(x) curves for different pressures are limited by recommended
%limitation of 20% in contraction percentage for the used PAM actuator
%(L = 260mm D=20mm)
function F1 = FxPmodel(P1,x_muscle1)
%Input: P comming from proporcional controller  is in bar. Its 6x1 vector
% x_muscle (in % contraction)
%Output:F according to P input and and x value of half of the maximun
%permissible stroke
%Importing 2 variable F(x,P) model
curve = @(x,P)  -0.002697-93.8*x+2.917*P+13.05*x^2-0.04264*x*P-0.001793*P^2-0.9395*x^3-0.001597*x^2*P-0.0001142*x*P^2+4.694e-06*P^3+0.03335*x^4+6.106e-06*x^3*P+2.699e-06*x^2*P^2+1.25e-07*x*P^3-5.675e-09*P^4-0.0004611*x^5+9.334e-07*x^4*P-1.221e-08*x^3*P^2-1.463e-09*x^2*P^3-4.929e-11*x*P^4+2.492e-12*P^5;
%Defining F and x vectors for the 6 actuators
F1 = zeros(length(P1),1); %6x1
x1 = zeros(length(P1),1); %6x1
% Transform P from bar to Kpa
P1 = 100*P1;

for i=1:length(P1)
% Obtaining the stroke
x1(i) = x_muscle1(i); 
% Obtaining the applied force
F1(i) = curve(x1(i),P1(i)); 
if F1(i)<0
    F1(i) = 0;
end
end
end

== matlab function walkingRobotRL3D/Walking Robot33/DYNAMIC MODEL OF PAM FOR RIGHT LEG/Dynamic Model Antagonisitic PAM2/F(x,P) mode (Muscles 1)1 ==
  data: P2 input; F2 output; x_muscle2 input
%Author: Eduardo Reyero Ibáñez
%Note: F(x) curves for different pressures are limited by recommended
%limitation of 20% in contraction percentage for the used PAM actuator
%(L = 260mm D=20mm)
function F2 = FxPmodel(P2,x_muscle2)
%Input: P comming from proporcional controller  is in bar. Its 6x1 vector
% x_muscle (in % contraction)
%Output:F according to P input and and x value of half of the maximun
%permissible stroke
%Importing 2 variable F(x,P) model
curve = @(x,P)  -0.002697-93.8*x+2.917*P+13.05*x^2-0.04264*x*P-0.001793*P^2-0.9395*x^3-0.001597*x^2*P-0.0001142*x*P^2+4.694e-06*P^3+0.03335*x^4+6.106e-06*x^3*P+2.699e-06*x^2*P^2+1.25e-07*x*P^3-5.675e-09*P^4-0.0004611*x^5+9.334e-07*x^4*P-1.221e-08*x^3*P^2-1.463e-09*x^2*P^3-4.929e-11*x*P^4+2.492e-12*P^5;
%Defining F and x vectors for the 6 actuators
F2 = zeros(length(P2),1); %6x1
x2 = zeros(length(P2),1); %6x1
% Transform P from bar to Kpa
P2 = 100*P2;

for i=1:length(P2)
% Obtaining the stroke
x2(i) = x_muscle2(i); 
% Obtaining the applied force
F2(i) = curve(x2(i),P2(i));
if F2(i)<0
    F2(i) = 0;
end
end
end

== matlab function walkingRobotRL3D/Walking Robot (Angle based)/Dynamic model of antagonistic PAM actuators/Proportional Regulator (Muscles 1) ==
  data: V1 input; reg_type input; p1 output
% Author: Eduardo Reyero Ibáñez
% Descrition: In this file it will be implemented the required input for the PAM
function p1  = propReg(V1,reg_type)
%% Proportional pressure regulators VPPM
%Range of Voltage
minVoltage = 0;
maxVoltage = 7.98; % This voltage provide 8 bar of pressure with regulator type 1
p1 = zeros(10,1);
%Initial pressure for muscles
%p1 = [1.764 0 1.764 1.764 0 1.764]';

%Select regulartor type
%reg_type = 1; % This will be given by the call of the function
%Limit the voltage
for i=1:length(p1)
if V1(i) >= maxVoltage 
    V1(i) = maxVoltage;
end
end
if reg_type == 1
    f_prop = @(V) 0.99*V+0.1;
    for i=1:length(p1)
    p1(i) = f_prop(V1(i));
    end
elseif reg_type == 2
    f_prop = @(V) 0.594*V+0.06;
    for i=1:length(p1)
    p1(i) = f_prop(V1(i));
    end
else
    f_prop = @(V) 0.198*V+0.02;
    for i=1:length(p1)
    p1(i) = f_prop(V1(i));
    end
end

% figure
% fplot(p1)
% xlim([0 10])
% ylim([0 10])
end

== matlab function walkingRobotRL3D/Walking Robot33/DYNAMIC MODEL OF PAM FOR RIGHT LEG/Dynamic Model Antagonisitic PAM2/Proportional Regulator (Muscles 1) ==
  data: V1 input; reg_type input; p1 output
% Author: Eduardo Reyero Ibáñez
% Descrition: In this file it will be implemented the required input for the PAM
function p1  = propReg(V1,reg_type)
%% Proportional pressure regulators VPPM
%Range of Voltage
minVoltage = 0;
maxVoltage = 7.98; % This voltage provide 8 bar of pressure with regulator type 1
p1 = zeros(1,1);
%Select regulartor type
%reg_type = 1; % This will be given by the call of the function
%Limit the voltage
for i=1:length(p1)
if V1(i) >= maxVoltage 
    V1(i) = maxVoltage;
end
end
if reg_type == 1
    f_prop = @(V) 0.99*V+0.1;
    for i=1:length(p1)
    p1(i) = f_prop(V1(i));
    end
elseif reg_type == 2
    f_prop = @(V) 0.594*V+0.06;
    for i=1:length(p1)
    p1(i) = f_prop(V1(i));
    end
else
    f_prop = @(V) 0.198*V+0.02;
    for i=1:length(p1)
    p1(i) = f_prop(V1(i));
    end
end

% figure
% fplot(p1)
% xlim([0 10])
% ylim([0 10])
end

== matlab function walkingRobotRL3D/Walking Robot33/DYNAMIC MODEL OF PAM FOR RIGHT LEG/Dynamic Model Antagonisitic PAM2/Proportional Regulator (Muscles 2) ==
  data: V1 input; reg_type input; p1 output
% Author: Eduardo Reyero Ibáñez
% Descrition: In this file it will be implemented the required input for the PAM
function p1  = propReg(V1,reg_type)
%% Proportional pressure regulators VPPM
%Range of Voltage
minVoltage = 0;
maxVoltage = 7.98; % This voltage provide 8 bar of pressure with regulator type 1
p1 = zeros(1,1);
%Select regulartor type
%reg_type = 1; % This will be given by the call of the function
%Limit the voltage
for i=1:length(p1)
if V1(i) >= maxVoltage 
    V1(i) = maxVoltage;
end
end
if reg_type == 1
    f_prop = @(V) 0.99*V+0.1;
    for i=1:length(p1)
    p1(i) = f_prop(V1(i));
    end
elseif reg_type == 2
    f_prop = @(V) 0.594*V+0.06;
    for i=1:length(p1)
    p1(i) = f_prop(V1(i));
    end
else
    f_prop = @(V) 0.198*V+0.02;
    for i=1:length(p1)
    p1(i) = f_prop(V1(i));
    end
end

% figure
% fplot(p1)
% xlim([0 10])
% ylim([0 10])
end

== matlab function walkingRobotRL3D/Walking Robot33/DYNAMIC MODEL OF PAM FOR RIGHT LEG/Dynamic Model Antagonisitic PAM2/Spring and damping model/S(P),D(P) ==
  data: P1 input; S1 output; P2 input; D1 output; S2 output; D2 output
function [S1,D1,S2,D2] = getSpringDampingCoeff(P1,P2)
tau = 0.6;
% Spring and damping coeff for muscle 1
if P1>=0 && P1<=1
    S1 = 400;
    D1 = tau*S1;
elseif P1>1 && P1<=2
    S1 = 500;
    D1 = tau*S1;
elseif P1>2 && P1<=3
    S1 = 1100;
    D1 = tau*S1;
elseif P1>3 && P1<=4
    S1 = 1500;
    D1 = tau*S1;
elseif P1>4 && P1<=5
    S1 = 2000;
    D1 = tau*S1;
elseif P1>5 && P1<=6
    S1 = 2900;
    D1 = tau*S1;
elseif P1>6 && P1<=7
    S1 = 3800;
    D1 = tau*S1;
elseif P1>7 && P1<=8.5
    S1 = 5000;
    D1 = tau*S1;
else %Never will enter here
    S1 = 800;
    D1 = tau*S1;  
end

% Spring and damping coeff for muscle 1
if P2>=0 && P2<=1
    S2 = 400;
    D2 = tau*S2;
elseif P2>1 && P2<=2
    S2 = 500;
    D2 = tau*S2;
elseif P2>2 && P2<=3
    S2 = 1100;
    D2 = tau*S2;
elseif P2>3 && P2<=4
    S2 = 1500;
    D2 = tau*S2;
elseif P2>4 && P2<=5
    S2 = 2000;
    D2 = tau*S2;
elseif P2>5 && P2<=6
    S2 = 2900;
    D2 = tau*S2;
elseif P2>6 && P2<=7
    S2 = 3800;
    D2 = tau*S2;
elseif P2>7 && P2<=8.5
    S2 = 5000;
    D2 = tau*S2;
else %Never will enter here
    S2 = 800;
    D2 = tau*S2;  
end

end

== matlab function walkingRobotRL3D/Walking Robot33/DYNAMIC MODEL OF PAM FOR RIGHT LEG/Dynamic Model Antagonisitic PAM3/F(x,P) mode (Muscles 1) ==
  data: P1 input; F1 output; x_muscle1 input
%Author: Eduardo Reyero Ibáñez
%Note: F(x) curves for different pressures are limited by recommended
%limitation of 20% in contraction percentage for the used PAM actuator
%(L = 260mm D=20mm)
function F1 = FxPmodel(P1,x_muscle1)
%Input: P comming from proporcional controller  is in bar. Its 6x1 vector
% x_muscle (in % contraction)
%Output:F according to P input and and x value of half of the maximun
%permissible stroke
%Importing 2 variable F(x,P) model
curve = @(x,P)  -0.002697-93.8*x+2.917*P+13.05*x^2-0.04264*x*P-0.001793*P^2-0.9395*x^3-0.001597*x^2*P-0.0001142*x*P^2+4.694e-06*P^3+0.03335*x^4+6.106e-06*x^3*P+2.699e-06*x^2*P^2+1.25e-07*x*P^3-5.675e-09*P^4-0.0004611*x^5+9.334e-07*x^4*P-1.221e-08*x^3*P^2-1.463e-09*x^2*P^3-4.929e-11*x*P^4+2.492e-12*P^5;
%Defining F and x vectors for the 6 actuators
F1 = zeros(length(P1),1); %6x1
x1 = zeros(length(P1),1); %6x1
% Transform P from bar to Kpa
P1 = 100*P1;

for i=1:length(P1)
% Obtaining the stroke
x1(i) = x_muscle1(i); 
% Obtaining the applied force
F1(i) = curve(x1(i),P1(i)); 
if F1(i)<0
    F1(i) = 0;
end
end
end

== matlab function walkingRobotRL3D/Walking Robot33/DYNAMIC MODEL OF PAM FOR RIGHT LEG/Dynamic Model Antagonisitic PAM3/F(x,P) mode (Muscles 1)1 ==
  data: P2 input; F2 output; x_muscle2 input
%Author: Eduardo Reyero Ibáñez
%Note: F(x) curves for different pressures are limited by recommended
%limitation of 20% in contraction percentage for the used PAM actuator
%(L = 260mm D=20mm)
function F2 = FxPmodel(P2,x_muscle2)
%Input: P comming from proporcional controller  is in bar. Its 6x1 vector
% x_muscle (in % contraction)
%Output:F according to P input and and x value of half of the maximun
%permissible stroke
%Importing 2 variable F(x,P) model
curve = @(x,P)  -0.002697-93.8*x+2.917*P+13.05*x^2-0.04264*x*P-0.001793*P^2-0.9395*x^3-0.001597*x^2*P-0.0001142*x*P^2+4.694e-06*P^3+0.03335*x^4+6.106e-06*x^3*P+2.699e-06*x^2*P^2+1.25e-07*x*P^3-5.675e-09*P^4-0.0004611*x^5+9.334e-07*x^4*P-1.221e-08*x^3*P^2-1.463e-09*x^2*P^3-4.929e-11*x*P^4+2.492e-12*P^5;
%Defining F and x vectors for the 6 actuators
F2 = zeros(length(P2),1); %6x1
x2 = zeros(length(P2),1); %6x1
% Transform P from bar to Kpa
P2 = 100*P2;

for i=1:length(P2)
% Obtaining the stroke
x2(i) = x_muscle2(i); 
% Obtaining the applied force
F2(i) = curve(x2(i),P2(i));
if F2(i)<0
    F2(i) = 0;
end
end
end

== matlab function walkingRobotRL3D/Walking Robot33/DYNAMIC MODEL OF PAM FOR RIGHT LEG/Dynamic Model Antagonisitic PAM3/Proportional Regulator (Muscles 1) ==
  data: V1 input; reg_type input; p1 output
% Author: Eduardo Reyero Ibáñez
% Descrition: In this file it will be implemented the required input for the PAM
function p1  = propReg(V1,reg_type)
%% Proportional pressure regulators VPPM
%Range of Voltage
minVoltage = 0;
maxVoltage = 7.98; % This voltage provide 8 bar of pressure with regulator type 1
p1 = zeros(1,1);
%Select regulartor type
%reg_type = 1; % This will be given by the call of the function
%Limit the voltage
for i=1:length(p1)
if V1(i) >= maxVoltage 
    V1(i) = maxVoltage;
end
end
if reg_type == 1
    f_prop = @(V) 0.99*V+0.1;
    for i=1:length(p1)
    p1(i) = f_prop(V1(i));
    end
elseif reg_type == 2
    f_prop = @(V) 0.594*V+0.06;
    for i=1:length(p1)
    p1(i) = f_prop(V1(i));
    end
else
    f_prop = @(V) 0.198*V+0.02;
    for i=1:length(p1)
    p1(i) = f_prop(V1(i));
    end
end

% figure
% fplot(p1)
% xlim([0 10])
% ylim([0 10])
end

== matlab function walkingRobotRL3D/Walking Robot33/DYNAMIC MODEL OF PAM FOR RIGHT LEG/Dynamic Model Antagonisitic PAM3/Proportional Regulator (Muscles 2) ==
  data: V1 input; reg_type input; p1 output
% Author: Eduardo Reyero Ibáñez
% Descrition: In this file it will be implemented the required input for the PAM
function p1  = propReg(V1,reg_type)
%% Proportional pressure regulators VPPM
%Range of Voltage
minVoltage = 0;
maxVoltage = 7.98; % This voltage provide 8 bar of pressure with regulator type 1
p1 = zeros(1,1);
%Select regulartor type
%reg_type = 1; % This will be given by the call of the function
%Limit the voltage
for i=1:length(p1)
if V1(i) >= maxVoltage 
    V1(i) = maxVoltage;
end
end
if reg_type == 1
    f_prop = @(V) 0.99*V+0.1;
    for i=1:length(p1)
    p1(i) = f_prop(V1(i));
    end
elseif reg_type == 2
    f_prop = @(V) 0.594*V+0.06;
    for i=1:length(p1)
    p1(i) = f_prop(V1(i));
    end
else
    f_prop = @(V) 0.198*V+0.02;
    for i=1:length(p1)
    p1(i) = f_prop(V1(i));
    end
end

% figure
% fplot(p1)
% xlim([0 10])
% ylim([0 10])
end
